simulink model "mux_demux"  (R2021a)
settings: Solver=VariableStepAuto  StartTime=0.0  StopTime=10.0  RelTol=1e-3
libraries: simulink x2
settings Model: Creator=Aula  LastModifiedBy=Aula

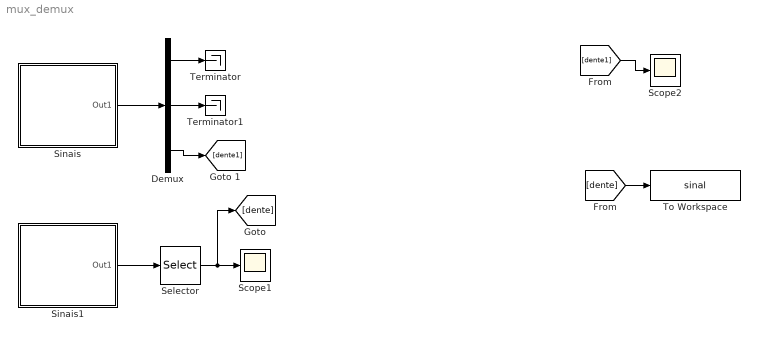
== system mux_demux ==
  Demux : Demux  Outputs=3
  Scope1 : Scope
  Scope2 : Scope
  Selector : Selector  InputPortWidth=3  IndexOptions=Index vector (dialog)  Indices=3  OutputSizes=1
  Sinais : Subsystem
  Sinais1 : Subsystem
  Terminator : Terminator
  Terminator1 : Terminator
  To Workspace : ToWorkspace  VariableName=sinal  SampleTime=0.1
  wires:
  Sinais/1(Out1) -> Demux/1
  Demux/1 -> Terminator/1
  Demux/2 -> Terminator1/1
  Sinais1/1(Out1) -> Selector/1
  Selector/1 -> [dente], Scope1/1
  [dente] -> To Workspace/1
  Demux/3 -> [dente1]
  [dente1] -> Scope2/1

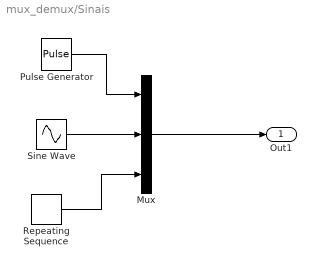
== system mux_demux/Sinais ==
  Mux : Mux  Inputs=3
  Pulse Generator : DiscretePulseGenerator  PulseType=Time based  PulseWidth=50
  Repeating Sequence : simulink/Sources/Repeating Sequence  rep_seq_t=[0 2]  rep_seq_y=[0 2]
  Sine Wave : Sin  SampleTime=0
  Out1 : Outport
  wires:
  Pulse Generator/1 -> Mux/1
  Repeating Sequence/1 -> Mux/3
  Sine Wave/1 -> Mux/2
  Mux/1 -> Out1/1

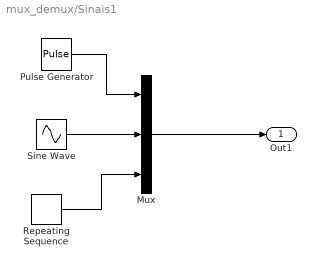
== system mux_demux/Sinais1 ==
  Mux : Mux  Inputs=3
  Pulse Generator : DiscretePulseGenerator  PulseType=Time based  PulseWidth=50
  Repeating Sequence : simulink/Sources/Repeating Sequence  rep_seq_t=[0 2]  rep_seq_y=[0 2]
  Sine Wave : Sin  SampleTime=0
  Out1 : Outport
  wires:
  Mux/1 -> Out1/1
  Sine Wave/1 -> Mux/2
  Repeating Sequence/1 -> Mux/3
  Pulse Generator/1 -> Mux/1
